simulink model "div"  (R2023a)
settings: Solver=FixedStepDiscrete  StartTime=0.0  StopTime=10.0  RelTol=1e-3
settings Model: DataTypeOverride=Off  Creator=jose.sanchez  LastModifiedBy=jose.sanchez
settings SolverCC: AlgebraicLoopSolver=TrustRegion
settings DataIOCC: LimitDataPoints=on  SaveOutput=off  SaveTime=off
settings OptimizationCC: BlockReduction=off  ConditionallyExecuteInputs=off  DefaultParameterBehavior=Inlined  LifeSpan=inf
settings DebuggingCC: AlgebraicLoopMsg=error  SingleTaskRateTransMsg=error  UnconnectedInputMsg=warning  UnconnectedOutputMsg=warning  UnconnectedLineMsg=warning  AllowSymbolicDim=off  StrictBusMsg=ErrorOnBusTreatedAsVector  SFUnexpectedBacktrackingDiag=warning  SFNoUnconditionalDefaultTransitionDiag=warning  SFExecutionAtInitializationDiag=none  ArithmeticOperatorsInVariantConditions=warning
settings HardwareCC: ProdBitPerPointer=32  ProdBitPerSizeT=32  ProdBitPerPtrDiffT=32  ProdLargestAtomicFloat=None  ProdIntDivRoundTo=Undefined  ProdEndianess=Unspecified  ProdWordSize=32  ProdHWDeviceType=ASIC/FPGA->ASIC/FPGA  ProdEqTarget=off
settings ModelReferenceCC: EnableRefExpFcnMdlSchedulingChecks=on
settings SFSimCC: SimUseLocalCustomCode=off  CustomCodeUndefinedFunction=UseInterfaceOnly
settings RTWCC: RTWUseLocalCustomCode=off
settings CodeAppCC: StateflowObjectComments=on
settings GRTTargetCC: TargetLangStandard=C89/C90 (ANSI)
settings ConfigComp: CovScope=ReferencedModels  CovMetricSettings=dw  CovSaveCumulativeToWorkspaceVar=on  CovSaveSingleToWorkspaceVar=on  CovExternalEMLEnable=off  CovSFcnEnable=off

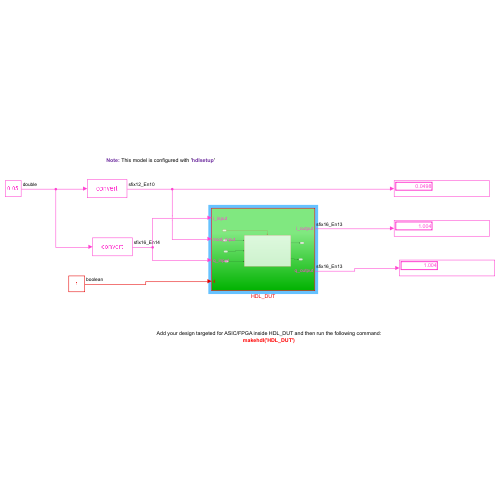
[thumbnail: Simulink's stored preview of the top-level diagram]
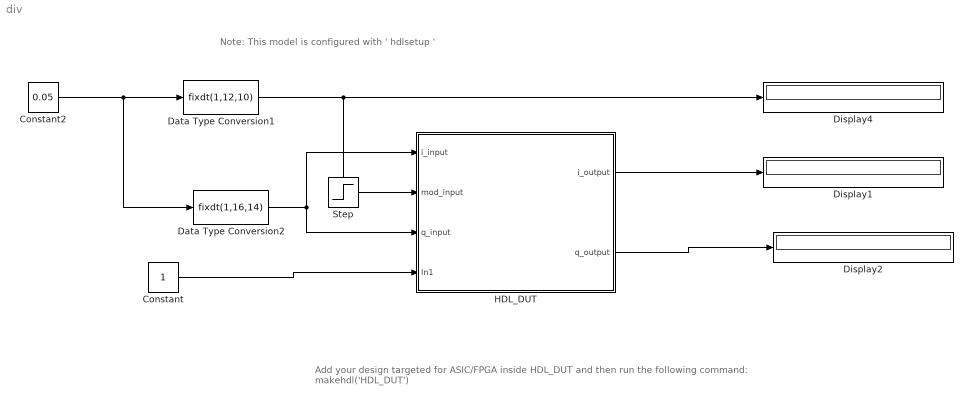
== system div ==
  note: Note: This model is configured with ' hdlsetup '
  note: Add your design targeted for ASIC/FPGA inside HDL_DUT and then run the following command:
      | makehdl('HDL_DUT')
  Constant : Constant  OutDataTypeStr=boolean  SampleTime=-1
  Constant2 : Constant  Value=0.05
  Data Type Conversion1 : DataTypeConversion  OutDataTypeStr=fixdt(1,12,10)  SaturateOnIntegerOverflow=off  RndMeth=Floor
  Data Type Conversion2 : DataTypeConversion  OutDataTypeStr=fixdt(1,16,14)  SaturateOnIntegerOverflow=off  RndMeth=Floor
  Display1 : Display
  Display2 : Display
  Display4 : Display
  HDL_DUT : Subsystem
  Step : Step  IOType=siggen  SampleTime=0
  wires:
  Data Type Conversion1/1 -> HDL_DUT/2(mod_input), Display4/1
  HDL_DUT/1(i_output) -> Display1/1
  HDL_DUT/2(q_output) -> Display2/1
  Constant2/1 -> Data Type Conversion2/1, Data Type Conversion1/1
  Data Type Conversion2/1 -> HDL_DUT/3(q_input), HDL_DUT/1(i_input)
  Constant/1 -> HDL_DUT/4(In1)

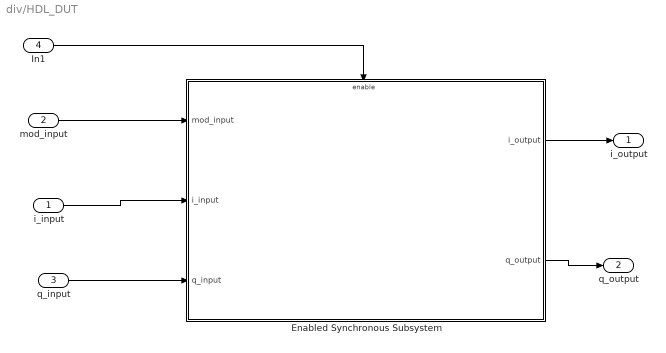
== system div/HDL_DUT ==
  i_input : Inport
  mod_input : Inport  Port=2
  q_input : Inport  Port=3
  In1 : Inport  Port=4
  Enabled Synchronous Subsystem : Subsystem  TreatAsAtomicUnit=on
  i_output : Outport  VectorParamsAs1DForOutWhenUnconnected=off
  q_output : Outport  Port=2  VectorParamsAs1DForOutWhenUnconnected=off
  wires:
  i_input/1 -> Enabled Synchronous Subsystem/2(i_input)
  q_input/1 -> Enabled Synchronous Subsystem/3(q_input)
  mod_input/1 -> Enabled Synchronous Subsystem/1(mod_input)
  Enabled Synchronous Subsystem/1(i_output) -> i_output/1
  Enabled Synchronous Subsystem/2(q_output) -> q_output/1
  In1/1 -> Enabled Synchronous Subsystem/Enable

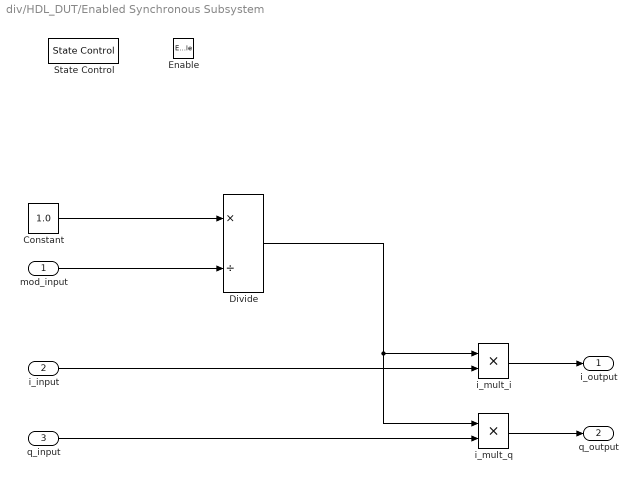
== system div/HDL_DUT/Enabled Synchronous Subsystem ==
  mod_input : Inport
  i_input : Inport  Port=2
  q_input : Inport  Port=3
  Enable : EnablePort
  Constant : Constant  Value=1.0  OutDataTypeStr=fixdt(1,20,18)
  Divide : Product  Inputs=*/  OutDataTypeStr=fixdt(1,20,8)  RndMeth=Zero  SaturateOnIntegerOverflow=on
  State Control : StateControl  StateControl=Synchronous
  i_mult_i : Product  Inputs=**  OutDataTypeStr=fixdt(1,16,13)  RndMeth=Zero  SaturateOnIntegerOverflow=on
  i_mult_q : Product  Inputs=**  OutDataTypeStr=fixdt(1,16,13)  RndMeth=Zero  SaturateOnIntegerOverflow=on
  i_output : Outport  VectorParamsAs1DForOutWhenUnconnected=off
  q_output : Outport  Port=2  VectorParamsAs1DForOutWhenUnconnected=off
  wires:
  i_input/1 -> i_mult_i/2
  Divide/1 -> i_mult_i/1, i_mult_q/1
  i_mult_i/1 -> i_output/1
  q_input/1 -> i_mult_q/2
  Constant/1 -> Divide/1
  mod_input/1 -> Divide/2
  i_mult_q/1 -> q_output/1
